simulink model "gm_sampleModel1879_1_sub"  (R2023a)
settings: Solver=VariableStepAuto  StartTime=0.0  StopTime=10.0  RelTol=1e-3
libraries: hdlsllib x2, simulink x1
settings Model: Creator=user1  LastModifiedBy=user1
settings OptimizationCC: BlockReduction=off  ConditionallyExecuteInputs=off
settings DebuggingCC: InheritedTsInSrcMsg=none

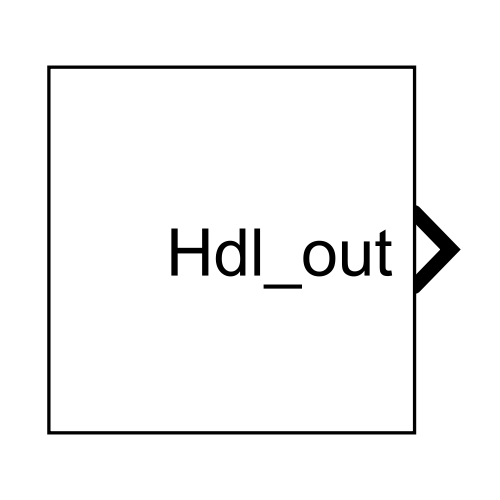
[thumbnail: Simulink's stored preview of the top-level diagram]
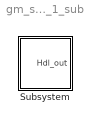
== system gm_sampleModel1879_1_sub ==
  Subsystem : Subsystem

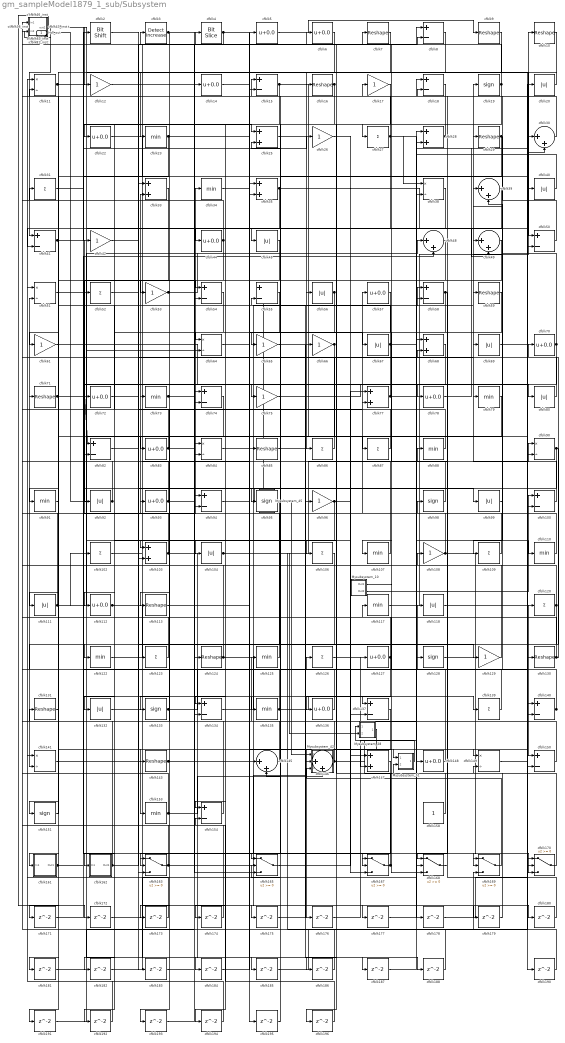
== system gm_sampleModel1879_1_sub/Subsystem ==
  Mysubsystem_10 : Subsystem
  Mysubsystem_28 : Subsystem
  Mysubsystem_42 : Subsystem
  Mysubsystem_45 : Subsystem
  Mysubsystem_51 : Subsystem
  cfblk{7,9..10,16,29,59,71,85,113,124,130..131,143} (13 alike) : Reshape
  cfblk{8,15,18,41,50,54..55,58,74,82,94,100,134,137,140,150,154} (17 alike) : Sum  Inputs=+-  OutDataTypeStr=uint8
  cfblk101_inst : Subsystem
  cfblk{27,31,52,86..87,102,106,109,120,123,126,139} (12 alike) : Sum  Inputs=+  OutDataTypeStr=uint8
  cfblk{25,28,33,35,68,77,103,147} (8 alike) : Sum  OutDataTypeStr=uint8
  cfblk{20,40,45,56,67,69,80,92,99,104,111,118,132} (13 alike) : Abs  OutDataTypeStr=uint8  SaturateOnIntegerOverflow=off
  cfblk{23,34,73,79,88,91,107,110,117,122,125,135,153} (13 alike) : MinMax  OutDataTypeStr=uint8
  cfblk{12,17,26,42,53,61,65..66,75,96,108,129} (12 alike) : Gain  OutDataTypeStr=uint8
  cfblk{11,38,51,64,84,90,141,149} (8 alike) : Product  Inputs=*/  OutDataTypeStr=uint8  RndMeth=Zero  SaturateOnIntegerOverflow=on
  cfblk{5..6,14,22,44,57,70,72,78,83,93,112,127,136,148} (15 alike) : Bias  Bias=0.0  SaturateOnIntegerOverflow=off
  cfblk114_inst : Subsystem
  cfblk116_inst : Subsystem
  cfblk121_inst : Subsystem
  cfblk{19,95,98,128,133,151} (6 alike) : Signum
  cfblk138_inst : Subsystem
  cfblk13_inst : Subsystem
  cfblk142_inst : Subsystem
  cfblk{30,39,48..49,145..146} (6 alike) : Sum  Inputs=|++  OutDataTypeStr=uint8
  cfblk158 : Constant  OutDataTypeStr=uint8  SampleTime=-1
  cfblk161 : Subsystem
  cfblk162 : Subsystem
  cfblk{163,165,167..170} (6 alike) : Switch  OutDataTypeStr=uint8  SaturateOnIntegerOverflow=off  InputSameDT=off
  cfblk{171..188,190..196} (25 alike) : Delay  SampleTime=1
  cfblk2 : hdlsllib/Logic and Bit Operations/Bit Shift  mode=Shift Left Logical  N=0
  cfblk21_inst : Subsystem
  cfblk3 : simulink/Logic and Bit Operations/Detect Increase  vinit=0.0  OutDataTypeStr=uint8
      settings: LibrarySourceBlock=|
      | hdlsllib/Logic and Bit
      | Operations/Detect
      | Increase
  cfblk36_inst : Subsystem
  cfblk4 : hdlsllib/Logic and Bit Operations/Bit Slice  lidx=7  ridx=0
  cfblk43_inst : Subsystem
  cfblk46_inst : Subsystem
  cfblk63_inst : Subsystem
  cfblk81_inst : Subsystem
  Hdl_out : Outport  OutDataTypeStr=uint8  SampleTime=1
  wires:
  Mysubsystem_10/1(Out1) -> cfblk168/3
  Mysubsystem_10/2(Out2) -> cfblk100/1
  Mysubsystem_28/1(Out1) -> cfblk176/1
  Mysubsystem_42/1(Out1) -> Mysubsystem_51/2(In2)
  Mysubsystem_45/1(y) -> cfblk55/1, Mysubsystem_42/1(In1)
  Mysubsystem_51/1(Out1) -> Mysubsystem_28/1(In1)
  cfblk10/1 -> cfblk86/1
  cfblk100/1 -> cfblk19/1
  cfblk101_inst/1(out1) -> cfblk46_inst/2(in2), cfblk184/1
  cfblk102/1 -> cfblk4/1
  cfblk103/1 -> cfblk33/2, cfblk185/1
  cfblk104/1 -> cfblk169/3, Mysubsystem_28/2(In2), cfblk79/1
  cfblk106/1 -> cfblk194/1
  cfblk107/1 -> cfblk63_inst/1(in1)
  cfblk108/1 -> cfblk81_inst/2(in2), cfblk57/1, cfblk170/3
  cfblk109/1 -> cfblk34/1
  cfblk11/1 -> cfblk83/1, cfblk44/1
  cfblk110/1 -> cfblk114_inst/1(in1)
  cfblk111/1 -> cfblk48/1, cfblk46_inst/1(in1), cfblk102/1
  cfblk112/1 -> cfblk14/1, cfblk188/1
  cfblk113/1 -> cfblk195/1
  cfblk114_inst/1(out1) -> Mysubsystem_45/1(In1)
  cfblk116_inst/1(out1) -> cfblk172/1
  cfblk117/1 -> cfblk10/1
  cfblk118/1 -> cfblk150/1
  cfblk12/1 -> cfblk124/1
  cfblk120/1 -> cfblk13_inst/1(in1), cfblk141/2
  cfblk121_inst/1(out1) -> cfblk127/1
  cfblk122/1 -> cfblk35/1
  cfblk123/1 -> cfblk138_inst/1(in1)
  cfblk124/1 -> cfblk33/1, cfblk170/2
  cfblk125/1 -> cfblk42/1
  cfblk126/1 -> cfblk178/1
  cfblk127/1 -> cfblk43_inst/1(in1), cfblk196/1
  cfblk128/1 -> cfblk170/1
  cfblk129/1 -> cfblk108/1
  cfblk13_inst/1(out1) -> cfblk123/1
  cfblk130/1 -> cfblk70/1, cfblk36_inst/1(in1)
  cfblk131/1 -> cfblk191/1
  cfblk132/1 -> cfblk175/1
  cfblk133/1 -> cfblk30/2, cfblk118/1
  cfblk134/1 -> cfblk58/1
  cfblk135/1 -> cfblk21_inst/2(in2), cfblk137/1, cfblk116_inst/2(in2)
  cfblk136/1 -> cfblk73/1
  cfblk137/1 -> cfblk171/1
  cfblk138_inst/1(out1) -> cfblk12/1
  cfblk139/1 -> cfblk88/1
  cfblk14/1 -> cfblk145/1
  cfblk140/1 -> cfblk49/1, cfblk51/2
  cfblk141/1 -> cfblk153/1
  cfblk142_inst/1(out1) -> cfblk50/1, cfblk41/1
  cfblk143/1 -> cfblk5/1, cfblk169/2
  cfblk145/1 -> cfblk125/1
  cfblk146/1 -> cfblk68/1, cfblk116_inst/1(in1)
  cfblk147/1 -> cfblk163/2
  cfblk148/1 -> cfblk117/1
  cfblk149/1 -> cfblk120/1
  cfblk15/1 -> cfblk190/1, cfblk162/1(In1)
  cfblk150/1 -> cfblk25/2
  cfblk151/1 -> cfblk11/2
  cfblk153/1 -> cfblk63_inst/2(in2), cfblk146/2
  cfblk154/1 -> cfblk93/1
  cfblk158/1 -> cfblk81_inst/1(in1)
  cfblk16/1 -> cfblk45/1, cfblk193/1
  cfblk161/1(Out1) -> cfblk94/2, cfblk126/1
  cfblk162/1(Out1) -> cfblk69/1, cfblk131/1
  cfblk163/1 -> cfblk59/1, cfblk13_inst/2(in2), cfblk177/1
  cfblk165/1 -> cfblk77/1
  cfblk167/1 -> cfblk74/2, cfblk3/1
  cfblk168/1 -> cfblk98/1
  cfblk169/1 -> Mysubsystem_42/3(In3)
  cfblk17/1 -> cfblk154/1
  cfblk170/1 -> cfblk84/1
  cfblk171/1 -> cfblk48/2
  cfblk172/1 -> cfblk146/1
  cfblk173/1 -> cfblk51/1
  cfblk174/1 -> cfblk121_inst/2(in2)
  cfblk175/1 -> cfblk168/2
  cfblk176/1 -> cfblk58/2
  cfblk177/1 -> cfblk90/1
  cfblk178/1 -> cfblk50/2
  cfblk179/1 -> cfblk149/2
  cfblk18/1 -> cfblk136/1
  cfblk180/1 -> cfblk18/2
  cfblk181/1 -> cfblk134/2
  cfblk182/1 -> cfblk35/2
  cfblk183/1 -> cfblk8/2
  cfblk184/1 -> cfblk68/2
  cfblk185/1 -> cfblk140/2
  cfblk186/1 -> cfblk165/2
  cfblk187/1 -> cfblk28/2
  cfblk188/1 -> cfblk142_inst/2(in2)
  cfblk19/1 -> cfblk145/2, cfblk101_inst/1(in1), cfblk66/1
  cfblk190/1 -> cfblk43_inst/2(in2)
  cfblk191/1 -> cfblk54/2
  cfblk192/1 -> cfblk141/1
  cfblk193/1 -> cfblk77/2
  cfblk194/1 -> cfblk11/1
  cfblk195/1 -> cfblk55/2
  cfblk196/1 -> cfblk154/2
  cfblk2/1 -> cfblk75/1
  cfblk20/1 -> cfblk16/1
  cfblk21_inst/1(out1) -> cfblk140/1
  cfblk22/1 -> cfblk85/1
  cfblk23/1 -> cfblk181/1, cfblk180/1
  cfblk25/1 -> cfblk56/1
  cfblk26/1 -> cfblk137/2
  cfblk27/1 -> cfblk41/2, cfblk114_inst/2(in2), cfblk38/1, cfblk110/1
  cfblk28/1 -> cfblk22/1, cfblk27/1
  cfblk29/1 -> cfblk165/1, cfblk109/1
  cfblk3/1 -> cfblk94/1, cfblk49/2, cfblk103/1
  cfblk30/1 -> cfblk18/1
  cfblk31/1 -> cfblk2/1
  cfblk33/1 -> cfblk92/1
  cfblk34/1 -> cfblk67/1
  cfblk35/1 -> cfblk147/1, cfblk104/1, cfblk100/2
  cfblk36_inst/1(out1) -> cfblk40/1
  cfblk38/1 -> cfblk61/1
  cfblk39/1 -> cfblk173/1
  cfblk4/1 -> cfblk138_inst/2(in2), cfblk38/2
  cfblk40/1 -> cfblk28/1
  cfblk41/1 -> cfblk80/1, cfblk26/1
  cfblk42/1 -> cfblk183/1
  cfblk43_inst/1(out1) -> cfblk139/1
  cfblk44/1 -> cfblk21_inst/1(in1), cfblk113/1, cfblk103/2
  cfblk45/1 -> cfblk192/1
  cfblk46_inst/1(out1) -> cfblk99/1, cfblk167/2
  cfblk48/1 -> cfblk91/1
  cfblk49/1 -> cfblk186/1
  cfblk5/1 -> cfblk9/1
  cfblk50/1 -> cfblk17/1
  cfblk51/1 -> cfblk53/1
  cfblk52/1 -> cfblk8/1
  cfblk53/1 -> cfblk29/1, cfblk165/3
  cfblk54/1 -> cfblk143/1
  cfblk55/1 -> cfblk65/1
  cfblk56/1 -> cfblk132/1, cfblk64/1, cfblk174/1
  cfblk57/1 -> cfblk84/2
  cfblk58/1 -> cfblk168/1, cfblk147/2
  cfblk59/1 -> cfblk107/1
  cfblk6/1 -> cfblk23/1
  cfblk61/1 -> cfblk96/1
  cfblk63_inst/1(out1) -> cfblk25/1
  cfblk64/1 -> Mysubsystem_51/1(In1)
  cfblk65/1 -> cfblk149/1
  cfblk66/1 -> cfblk163/1, cfblk182/1
  cfblk67/1 -> cfblk150/2, cfblk106/1, cfblk31/1
  cfblk68/1 -> cfblk87/1
  cfblk69/1 -> cfblk20/1
  cfblk7/1 -> cfblk133/1
  cfblk70/1 -> cfblk39/2, cfblk134/1
  cfblk71/1 -> cfblk82/1, cfblk128/1, cfblk64/2, Mysubsystem_42/2(In2)
  cfblk72/1 -> cfblk129/1
  cfblk73/1 -> cfblk95/1, cfblk169/1
  cfblk74/1 -> cfblk161/1(In1)
  cfblk75/1 -> cfblk78/1
  cfblk77/1 -> cfblk72/1, cfblk148/1, cfblk90/2
  cfblk78/1 -> cfblk30/1
  cfblk79/1 -> cfblk82/2
  cfblk8/1 -> cfblk111/1
  cfblk80/1 -> cfblk101_inst/2(in2)
  cfblk81_inst/1(out1) -> cfblk54/1
  cfblk82/1 -> cfblk74/1
  cfblk83/1 -> cfblk36_inst/2(in2), cfblk135/1
  cfblk84/1 -> cfblk6/1
  cfblk85/1 -> cfblk187/1
  cfblk86/1 -> cfblk15/1
  cfblk87/1 -> cfblk142_inst/1(in1)
  cfblk88/1 -> cfblk52/1
  cfblk9/1 -> cfblk15/2
  cfblk90/1 -> cfblk163/3, cfblk130/1
  cfblk91/1 -> cfblk151/1
  cfblk92/1 -> cfblk71/1, Hdl_out/1
  cfblk93/1 -> cfblk167/1, cfblk121_inst/1(in1)
  cfblk94/1 -> cfblk179/1
  cfblk95/1 -> cfblk122/1
  cfblk96/1 -> cfblk167/3, cfblk112/1
  cfblk98/1 -> cfblk7/1
  cfblk99/1 -> cfblk39/1

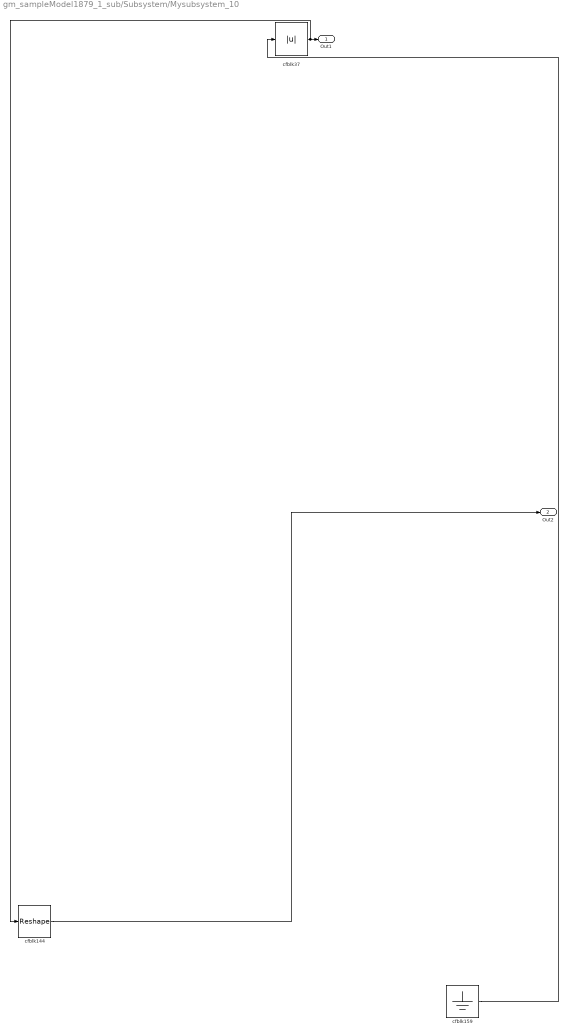
== system gm_sampleModel1879_1_sub/Subsystem/Mysubsystem_10 ==
  cfblk144 : Reshape
  cfblk159 : Ground
  cfblk37 : Abs  SaturateOnIntegerOverflow=off
  Out1 : Outport  SampleTime=1
  Out2 : Outport  Port=2  SampleTime=1
  wires:
  cfblk144/1 -> Out2/1
  cfblk159/1 -> cfblk37/1
  cfblk37/1 -> cfblk144/1, Out1/1

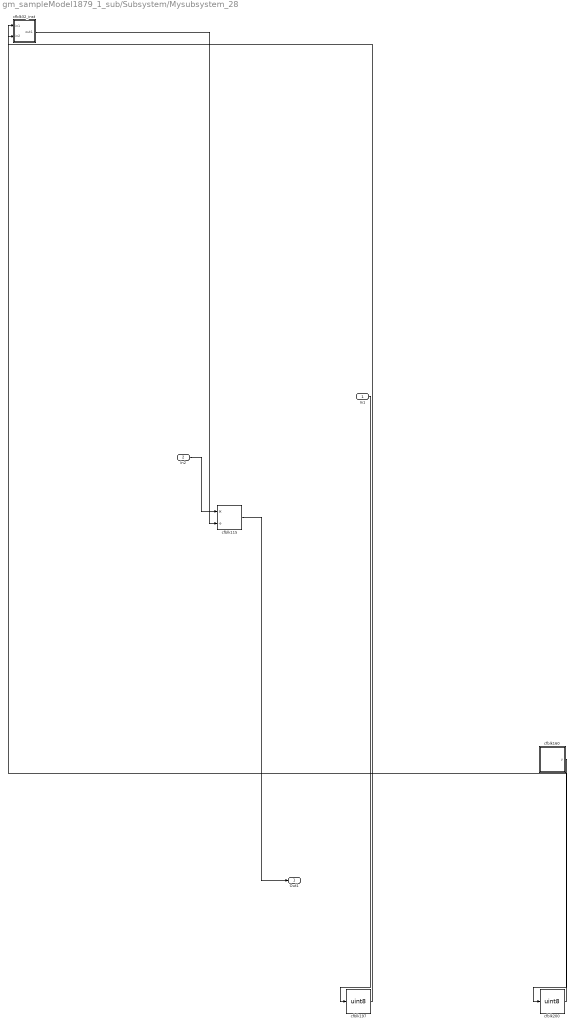
== system gm_sampleModel1879_1_sub/Subsystem/Mysubsystem_28 ==
  In1 : Inport  OutDataTypeStr=uint8  PortDimensions=1  SampleTime=1
  In2 : Inport  Port=2  OutDataTypeStr=uint8  PortDimensions=1  SampleTime=1
  cfblk115 : Product  Inputs=*/  RndMeth=Zero  SaturateOnIntegerOverflow=on
  cfblk160 : Subsystem  mask(Counter Free-Running){NumBits=double(16), tsamp=double(-1)}
      mask prompts: NumBits "Simulink:masks:NumberOfBits_MP"; tsamp "Simulink:masks:SampleTime_MP"
      mask help: Simulink:masks:CounterFreeRunning_MD
  cfblk197 : DataTypeConversion  OutDataTypeStr=uint8  SaturateOnIntegerOverflow=off  RndMeth=Floor
  cfblk200 : DataTypeConversion  OutDataTypeStr=uint8  SaturateOnIntegerOverflow=off  RndMeth=Floor
  cfblk32_inst : Subsystem
  Out1 : Outport  SampleTime=1
  wires:
  In1/1 -> cfblk197/1
  In2/1 -> cfblk115/1
  cfblk115/1 -> Out1/1
  cfblk160/1(y) -> cfblk200/1
  cfblk197/1 -> cfblk32_inst/1(in1)
  cfblk200/1 -> cfblk32_inst/2(in2)
  cfblk32_inst/1(out1) -> cfblk115/2

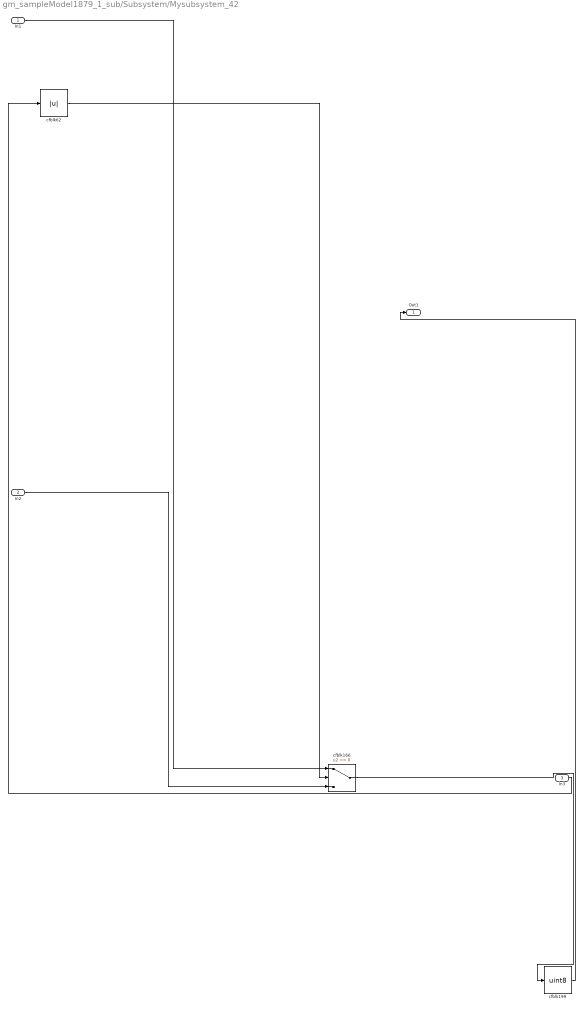
== system gm_sampleModel1879_1_sub/Subsystem/Mysubsystem_42 ==
  In1 : Inport  OutDataTypeStr=boolean  PortDimensions=1  SampleTime=1
  In2 : Inport  Port=2  OutDataTypeStr=uint8  PortDimensions=1  SampleTime=1
  In3 : Inport  Port=3  OutDataTypeStr=uint8  PortDimensions=1  SampleTime=1
  cfblk166 : Switch  SaturateOnIntegerOverflow=off  InputSameDT=off
  cfblk199 : DataTypeConversion  OutDataTypeStr=uint8  SaturateOnIntegerOverflow=off  RndMeth=Floor
  cfblk62 : Abs  SaturateOnIntegerOverflow=off
  Out1 : Outport  SampleTime=1
  wires:
  In1/1 -> cfblk166/1
  In2/1 -> cfblk166/3
  In3/1 -> cfblk62/1
  cfblk166/1 -> cfblk199/1
  cfblk199/1 -> Out1/1
  cfblk62/1 -> cfblk166/2

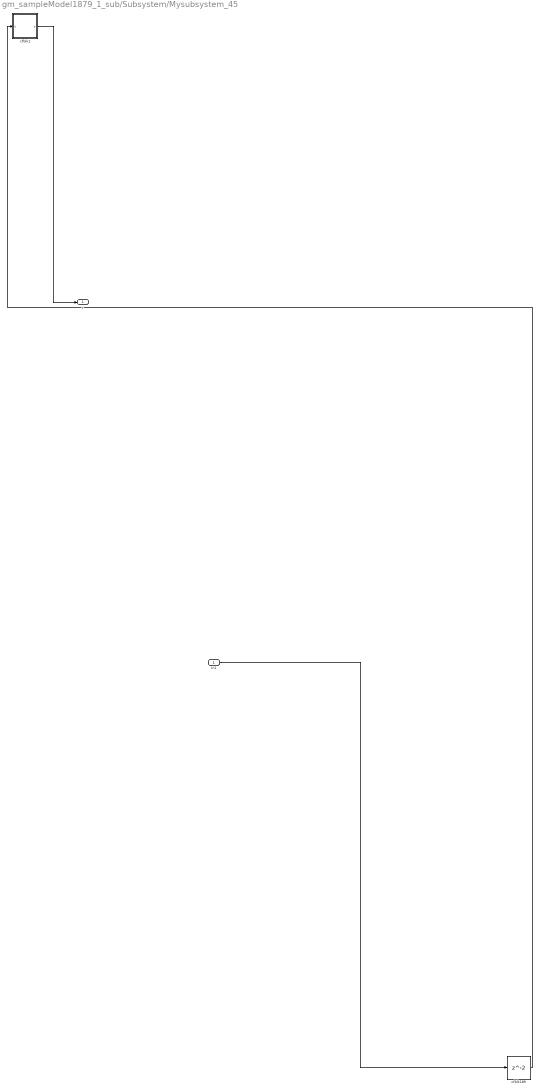
== system gm_sampleModel1879_1_sub/Subsystem/Mysubsystem_45 ==
  In1 : Inport  OutDataTypeStr=uint8  PortDimensions=1  SampleTime=1
  cfblk1 : Subsystem  mask(Compare To Constant){relop=<=, const=double(3), OutDataTypeStr=boolean, ZeroCross=on}
      mask prompts: relop "Simulink:masks:Operator_MP"; const "Simulink:masks:ConstantValue_MP"; OutDataTypeStr "Simulink:masks:OutputDataType_MP"; ZeroCross "Simulink:masks:EnableZerocrossingDetection_MP"
      mask help: Simulink:masks:CompareToConstant_MD
      mask init:
      | OutDataTypeStr = 'boolean';
      | ZeroCross = 'on';
      | blkName = 'sampleModel1879_1_sub/Subsystem/Mysubsystem_45/cfblk1';
      | const = double(3);
      | const_str = '3.0';
      | const_val = double(3);
      | relop = '<=';
      | setValue = 'boolean';
      | str = '<= 3';
      mask TypeOptions relop: == | ~= | < | <= | >= | >
      mask TypeOptions OutDataTypeStr: Simulink:masks:uint8 | Simulink:masks:boolean
      mask Callback ZeroCross: sl('zeroCrossEnable', gcbh);
      mask Display: disp(str)
  cfblk189 : Delay  SampleTime=1
  y : Outport  SampleTime=1
  wires:
  In1/1 -> cfblk189/1
  cfblk1/1(y) -> y/1
  cfblk189/1 -> cfblk1/1(u)

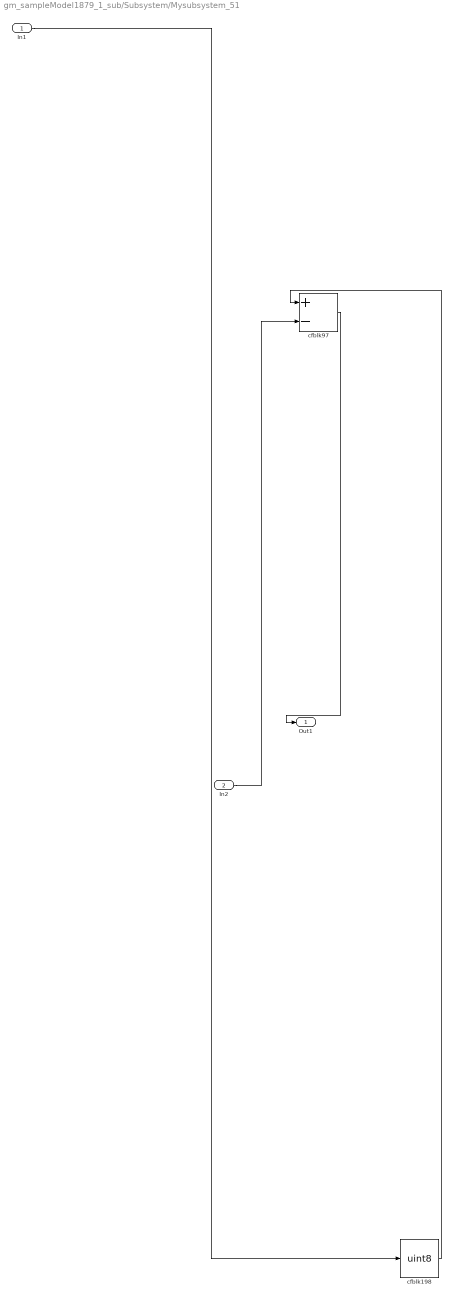
== system gm_sampleModel1879_1_sub/Subsystem/Mysubsystem_51 ==
  In1 : Inport  OutDataTypeStr=uint8  PortDimensions=1  SampleTime=1
  In2 : Inport  Port=2  OutDataTypeStr=uint8  PortDimensions=1  SampleTime=1
  cfblk198 : DataTypeConversion  OutDataTypeStr=uint8  SaturateOnIntegerOverflow=off  RndMeth=Floor
  cfblk97 : Sum  Inputs=+-
  Out1 : Outport  SampleTime=1
  wires:
  In1/1 -> cfblk198/1
  In2/1 -> cfblk97/2
  cfblk198/1 -> cfblk97/1
  cfblk97/1 -> Out1/1

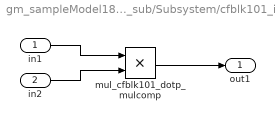
== system gm_sampleModel1879_1_sub/Subsystem/cfblk101_inst ==
  in1 : Inport  OutDataTypeStr=uint8  SampleTime=1
  in2 : Inport  Port=2  OutDataTypeStr=uint8  SampleTime=1
  mul_cfblk101_dotp_mulcomp : Product  Inputs=**  OutDataTypeStr=uint8  SampleTime=1
  out1 : Outport  OutDataTypeStr=uint8  SampleTime=1
  wires:
  in1/1 -> mul_cfblk101_dotp_mulcomp/1
  in2/1 -> mul_cfblk101_dotp_mulcomp/2
  mul_cfblk101_dotp_mulcomp/1 -> out1/1

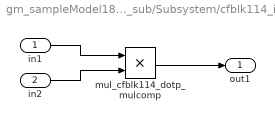
== system gm_sampleModel1879_1_sub/Subsystem/cfblk114_inst ==
  in1 : Inport  OutDataTypeStr=uint8  SampleTime=1
  in2 : Inport  Port=2  OutDataTypeStr=uint8  SampleTime=1
  mul_cfblk114_dotp_mulcomp : Product  Inputs=**  OutDataTypeStr=uint8  SampleTime=1
  out1 : Outport  OutDataTypeStr=uint8  SampleTime=1
  wires:
  in1/1 -> mul_cfblk114_dotp_mulcomp/1
  in2/1 -> mul_cfblk114_dotp_mulcomp/2
  mul_cfblk114_dotp_mulcomp/1 -> out1/1

== system gm_sampleModel1879_1_sub/Subsystem/cfblk116_inst ==
  in1 : Inport  OutDataTypeStr=uint8  SampleTime=1
  in2 : Inport  Port=2  OutDataTypeStr=uint8  SampleTime=1
  mul_cfblk116_dotp_mulcomp : Product  Inputs=**  OutDataTypeStr=uint8  SampleTime=1
  out1 : Outport  OutDataTypeStr=uint8  SampleTime=1
  wires:
  in1/1 -> mul_cfblk116_dotp_mulcomp/1
  in2/1 -> mul_cfblk116_dotp_mulcomp/2
  mul_cfblk116_dotp_mulcomp/1 -> out1/1

== system gm_sampleModel1879_1_sub/Subsystem/cfblk121_inst ==
  in1 : Inport  OutDataTypeStr=uint8  SampleTime=1
  in2 : Inport  Port=2  OutDataTypeStr=uint8  SampleTime=1
  mul_cfblk121_dotp_mulcomp : Product  Inputs=**  OutDataTypeStr=uint8  SampleTime=1
  out1 : Outport  OutDataTypeStr=uint8  SampleTime=1
  wires:
  in1/1 -> mul_cfblk121_dotp_mulcomp/1
  in2/1 -> mul_cfblk121_dotp_mulcomp/2
  mul_cfblk121_dotp_mulcomp/1 -> out1/1

== system gm_sampleModel1879_1_sub/Subsystem/cfblk138_inst ==
  in1 : Inport  OutDataTypeStr=uint8  SampleTime=1
  in2 : Inport  Port=2  OutDataTypeStr=uint8  SampleTime=1
  mul_cfblk138_dotp_mulcomp : Product  Inputs=**  OutDataTypeStr=uint8  SampleTime=1
  out1 : Outport  OutDataTypeStr=uint8  SampleTime=1
  wires:
  in1/1 -> mul_cfblk138_dotp_mulcomp/1
  in2/1 -> mul_cfblk138_dotp_mulcomp/2
  mul_cfblk138_dotp_mulcomp/1 -> out1/1

== system gm_sampleModel1879_1_sub/Subsystem/cfblk13_inst ==
  in1 : Inport  OutDataTypeStr=uint8  SampleTime=1
  in2 : Inport  Port=2  OutDataTypeStr=uint8  SampleTime=1
  mul_cfblk13_dotp_mulcomp : Product  Inputs=**  OutDataTypeStr=uint8  SampleTime=1
  out1 : Outport  OutDataTypeStr=uint8  SampleTime=1
  wires:
  in1/1 -> mul_cfblk13_dotp_mulcomp/1
  in2/1 -> mul_cfblk13_dotp_mulcomp/2
  mul_cfblk13_dotp_mulcomp/1 -> out1/1

== system gm_sampleModel1879_1_sub/Subsystem/cfblk142_inst ==
  in1 : Inport  OutDataTypeStr=uint8  SampleTime=1
  in2 : Inport  Port=2  OutDataTypeStr=uint8  SampleTime=1
  mul_cfblk142_dotp_mulcomp : Product  Inputs=**  OutDataTypeStr=uint8  SampleTime=1
  out1 : Outport  OutDataTypeStr=uint8  SampleTime=1
  wires:
  in1/1 -> mul_cfblk142_dotp_mulcomp/1
  in2/1 -> mul_cfblk142_dotp_mulcomp/2
  mul_cfblk142_dotp_mulcomp/1 -> out1/1

== system gm_sampleModel1879_1_sub/Subsystem/cfblk161 ==
  In1 : Inport  OutDataTypeStr=uint8  PortDimensions=1  SampleTime=1
  Out1 : Outport  SampleTime=1
  wires:
  In1/1 -> Out1/1

== system gm_sampleModel1879_1_sub/Subsystem/cfblk162 ==
  In1 : Inport  OutDataTypeStr=uint8  PortDimensions=1  SampleTime=1
  Out1 : Outport  SampleTime=1
  wires:
  In1/1 -> Out1/1

== system gm_sampleModel1879_1_sub/Subsystem/cfblk21_inst ==
  in1 : Inport  OutDataTypeStr=uint8  SampleTime=1
  in2 : Inport  Port=2  OutDataTypeStr=uint8  SampleTime=1
  mul_cfblk21_dotp_mulcomp : Product  Inputs=**  OutDataTypeStr=uint8  SampleTime=1
  out1 : Outport  OutDataTypeStr=uint8  SampleTime=1
  wires:
  in1/1 -> mul_cfblk21_dotp_mulcomp/1
  in2/1 -> mul_cfblk21_dotp_mulcomp/2
  mul_cfblk21_dotp_mulcomp/1 -> out1/1

== system gm_sampleModel1879_1_sub/Subsystem/cfblk36_inst ==
  in1 : Inport  OutDataTypeStr=uint8  SampleTime=1
  in2 : Inport  Port=2  OutDataTypeStr=uint8  SampleTime=1
  mul_cfblk36_dotp_mulcomp : Product  Inputs=**  OutDataTypeStr=uint8  SampleTime=1
  out1 : Outport  OutDataTypeStr=uint8  SampleTime=1
  wires:
  in1/1 -> mul_cfblk36_dotp_mulcomp/1
  in2/1 -> mul_cfblk36_dotp_mulcomp/2
  mul_cfblk36_dotp_mulcomp/1 -> out1/1

== system gm_sampleModel1879_1_sub/Subsystem/cfblk43_inst ==
  in1 : Inport  OutDataTypeStr=uint8  SampleTime=1
  in2 : Inport  Port=2  OutDataTypeStr=uint8  SampleTime=1
  mul_cfblk43_dotp_mulcomp : Product  Inputs=**  OutDataTypeStr=uint8  SampleTime=1
  out1 : Outport  OutDataTypeStr=uint8  SampleTime=1
  wires:
  in1/1 -> mul_cfblk43_dotp_mulcomp/1
  in2/1 -> mul_cfblk43_dotp_mulcomp/2
  mul_cfblk43_dotp_mulcomp/1 -> out1/1

== system gm_sampleModel1879_1_sub/Subsystem/cfblk46_inst ==
  in1 : Inport  OutDataTypeStr=uint8  SampleTime=1
  in2 : Inport  Port=2  OutDataTypeStr=uint8  SampleTime=1
  mul_cfblk46_dotp_mulcomp : Product  Inputs=**  OutDataTypeStr=uint8  SampleTime=1
  out1 : Outport  OutDataTypeStr=uint8  SampleTime=1
  wires:
  in1/1 -> mul_cfblk46_dotp_mulcomp/1
  in2/1 -> mul_cfblk46_dotp_mulcomp/2
  mul_cfblk46_dotp_mulcomp/1 -> out1/1

== system gm_sampleModel1879_1_sub/Subsystem/cfblk63_inst ==
  in1 : Inport  OutDataTypeStr=uint8  SampleTime=1
  in2 : Inport  Port=2  OutDataTypeStr=uint8  SampleTime=1
  mul_cfblk63_dotp_mulcomp : Product  Inputs=**  OutDataTypeStr=uint8  SampleTime=1
  out1 : Outport  OutDataTypeStr=uint8  SampleTime=1
  wires:
  in1/1 -> mul_cfblk63_dotp_mulcomp/1
  in2/1 -> mul_cfblk63_dotp_mulcomp/2
  mul_cfblk63_dotp_mulcomp/1 -> out1/1

== system gm_sampleModel1879_1_sub/Subsystem/cfblk81_inst ==
  in1 : Inport  OutDataTypeStr=uint8  SampleTime=1
  in2 : Inport  Port=2  OutDataTypeStr=uint8  SampleTime=1
  mul_cfblk81_dotp_mulcomp : Product  Inputs=**  OutDataTypeStr=uint8  SampleTime=1
  out1 : Outport  OutDataTypeStr=uint8  SampleTime=1
  wires:
  in1/1 -> mul_cfblk81_dotp_mulcomp/1
  in2/1 -> mul_cfblk81_dotp_mulcomp/2
  mul_cfblk81_dotp_mulcomp/1 -> out1/1

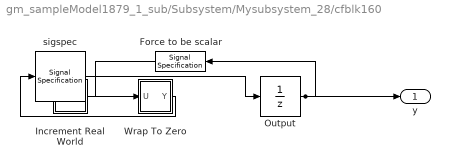
== system gm_sampleModel1879_1_sub/Subsystem/Mysubsystem_28/cfblk160 ==
  Force to be scalar : SignalSpecification  DisableCoverage=on  Dimensions=1
  Increment Real World : Subsystem  mask(Real World Value Increment){}
      mask help: Simulink:masks:RealWorldValueIncrement_MD
      mask Display: disp('V++')
  Output : UnitDelay  InitialCondition=0.0  SampleTime=tsamp  HasFrameUpgradeWarning=on
  Wrap To Zero : Subsystem  mask(Wrap To Zero){Threshold=double(65535)}
      mask prompts: Threshold "Simulink:masks:Threshold_MP"
      mask help: Simulink:masks:WrapToZero_MD
  sigspec : SignalSpecification  OutDataTypeStr=uint16  Dimensions=1
  y : Outport  SampleTime=1
  wires:
  Force to be scalar/1 -> Increment Real World/1(u)
  Increment Real World/1(y) -> Wrap To Zero/1(U)
  Output/1 -> Force to be scalar/1, y/1
  Wrap To Zero/1(Y) -> sigspec/1
  sigspec/1 -> Output/1

== system gm_sampleModel1879_1_sub/Subsystem/Mysubsystem_28/cfblk32_inst ==
  in1 : Inport  OutDataTypeStr=uint8  SampleTime=1
  in2 : Inport  Port=2  OutDataTypeStr=uint8  SampleTime=1
  mul_cfblk32_dotp_mulcomp : Product  Inputs=**  OutDataTypeStr=uint16  SampleTime=1
  out1 : Outport  OutDataTypeStr=uint16  SampleTime=1
  wires:
  in1/1 -> mul_cfblk32_dotp_mulcomp/1
  in2/1 -> mul_cfblk32_dotp_mulcomp/2
  mul_cfblk32_dotp_mulcomp/1 -> out1/1

== system gm_sampleModel1879_1_sub/Subsystem/Mysubsystem_45/cfblk1 ==
  u : Inport  OutDataTypeStr=uint8  SampleTime=1
  Compare : RelationalOperator  Operator=<=  OutDataTypeStr=boolean
  Constant : Constant  DisableCoverage=on  Value=const  OutDataTypeStr=Inherit: Inherit via back propagation  SampleTime=-1
  y : Outport  SampleTime=1
  wires:
  u/1 -> Compare/1
  Compare/1 -> y/1
  Constant/1 -> Compare/2

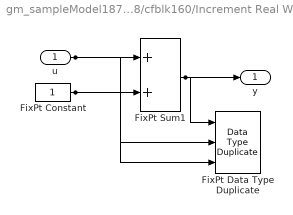
== system gm_sampleModel1879_1_sub/Subsystem/Mysubsystem_28/cfblk160/Increment Real World ==
  u : Inport  OutDataTypeStr=uint16  SampleTime=1
  FixPt Constant : Constant  DisableCoverage=on  OutDataTypeStr=Inherit: Inherit via back propagation  SampleTime=-1
  FixPt Data Type Duplicate : DataTypeDuplicate  DisableCoverage=on  NumInputPorts=3
  FixPt Sum1 : Sum  InputSameDT=on  OutDataTypeStr=Inherit: Inherit via back propagation  LockScale=on
  y : Outport  SampleTime=1
  wires:
  u/1 -> FixPt Sum1/1, FixPt Data Type Duplicate/2
  FixPt Constant/1 -> FixPt Sum1/2, FixPt Data Type Duplicate/3
  FixPt Sum1/1 -> FixPt Data Type Duplicate/1, y/1

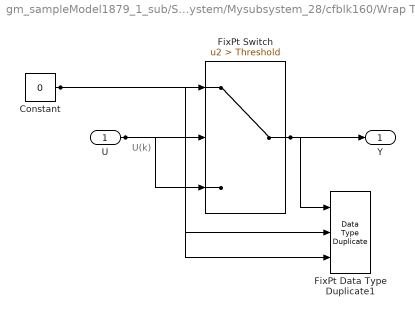
== system gm_sampleModel1879_1_sub/Subsystem/Mysubsystem_28/cfblk160/Wrap To Zero ==
  note: U(k)
  U : Inport  OutDataTypeStr=uint16  SampleTime=1
  Constant : Constant  DisableCoverage=on  Value=0  OutDataTypeStr=Inherit: Inherit via back propagation  SampleTime=-1
  FixPt Data Type Duplicate1 : DataTypeDuplicate  DisableCoverage=on  NumInputPorts=3
  FixPt Switch : Switch  Criteria=u2 > Threshold  Threshold=Threshold  OutDataTypeStr=Inherit: Inherit via back propagation  ZeroCross=off  SaturateOnIntegerOverflow=off  InputSameDT=off
  Y : Outport  SampleTime=1
  wires:
  U/1 -> FixPt Switch/3, FixPt Switch/2, FixPt Data Type Duplicate1/2
  Constant/1 -> FixPt Switch/1, FixPt Data Type Duplicate1/3
  FixPt Switch/1 -> FixPt Data Type Duplicate1/1, Y/1
